simulink model "trajgen_pos_raspberrypi"  (R2018b)
settings: Solver=FixedStepDiscrete  StartTime=0.0  StopTime=10.0  RelTol=1e-3  EnableMultiTasking=on
settings Model: Creator=ihout_000  LastModifiedBy=ihout
settings SolverCC: PositivePriorityOrder=on
settings DataIOCC: LimitDataPoints=on  SaveFormat=Array
settings OptimizationCC: EnhancedBackFolding=on  PassReuseOutputArgsAs=Individual arguments  ExpressionDepthLimit=2147483647  MaxStackSize=64  SimCompilerOptimization=on  OptimizeBlockOrder=speed  DifferentSizesBufferReuse=on  OptimizationCustomize=off
settings DebuggingCC: UnderspecifiedInitializationDetection=Classic  MergeDetectMultiDrivingBlocksExec=none  SolverPrmCheckMsg=warning  ParameterTunabilityLossMsg=error  StateNameClashWarn=warning  SFUnexpectedBacktrackingDiag=warning  SFNoUnconditionalDefaultTransitionDiag=warning  SFExecutionAtInitializationDiag=none
settings HardwareCC: ProdBitPerPointer=32  ProdBitPerSizeT=32  ProdBitPerPtrDiffT=32  ProdLargestAtomicInteger=Long  ProdLargestAtomicFloat=Double  ProdWordSize=32  ProdHWDeviceType=ARM Compatible->ARM Cortex  UseEmbeddedCoderFeatures=off  UseSimulinkCoderFeatures=off
settings ModelReferenceCC: PropagateSignalLabelsOutOfModel=off
settings SFSimCC: SimUserIncludeDirs=ReflexxesTypeII\include\  SimUseLocalCustomCode=off  MATLABDynamicMemAlloc=off
settings SFSimCC: SimUserSources=|
  | ReflexxesTypeII\src\TypeIIRML\ReflexxesAPI.cpp
  | ReflexxesTypeII\src\TypeIIRML\TypeIIRMLCalculatePositionalExtrems.cpp
  | ReflexxesTypeII\src\TypeIIRML\TypeIIRMLDecisions.cpp
  | ReflexxesTypeII\src\TypeIIRML\TypeIIRMLDecisionTree1A.cpp
  | ReflexxesTypeII\src\TypeIIRML\TypeIIRMLDecisionTree1B.cpp
  | ReflexxesTypeII\src\TypeIIRML\TypeIIRMLDecisionTree1C.cpp
  | ReflexxesTypeII\src\TypeIIRML\TypeIIRMLDecisionTree2.cpp
  | ReflexxesTypeII\src\TypeIIRML\TypeIIRMLFallBackStrategy.cpp
  | ReflexxesTypeII\src\TypeIIRML\TypeIIRMLIsPhaseSynchronizationPossible.cpp
  | ReflexxesTypeII\src\TypeIIRML\TypeIIRMLPolynomial.cpp
  | ReflexxesTypeII\src\TypeIIRML\TypeIIRMLPosition.cpp
  | ReflexxesTypeII\src\TypeIIRML\TypeIIRMLQuicksort.cpp
  | ReflexxesTypeII\src\TypeIIRML\TypeIIRMLSetupModifiedSelectionVector.cpp
  | ReflexxesTypeII\src\TypeIIRML\TypeIIRMLStep1.cpp
  | ReflexxesTypeII\src\TypeIIRML\TypeIIRMLStep1IntermediateProfiles.cpp
  | ReflexxesTypeII\src\TypeIIRML\TypeIIRMLStep1Profiles.cpp
  | ReflexxesTypeII\src\TypeIIRML\TypeIIRMLStep2.cpp
  | ReflexxesTypeII\src\TypeIIRML\TypeIIRMLStep2IntermediateProfiles.cpp
  | ReflexxesTypeII\src\TypeIIRML\TypeIIRMLStep2PhaseSynchronization.cpp
  | ReflexxesTypeII\src\TypeIIRML\TypeIIRMLStep2Profiles.cpp
  | ReflexxesTypeII\src\TypeIIRML\TypeIIRMLStep2WithoutSynchronization.cpp
  | ReflexxesTypeII\src\TypeIIRML\TypeIIRMLStep3.cpp
  | ReflexxesTypeII\src\TypeIIRML\TypeIIRMLVelocity.cpp
  | ReflexxesTypeII\src\TypeIIRML\TypeIIRMLVelocityCalculatePositionalExtrems.cpp
  | ReflexxesTypeII\src\TypeIIRML\TypeIIRMLVelocityFallBackStrategy.cpp
  | ReflexxesTypeII\src\TypeIIRML\TypeIIRMLVelocityIsPhaseSynchronizationPossible.cpp
  | ReflexxesTypeII\src\TypeIIRML\TypeIIRMLVelocityMethods.cpp
  | ReflexxesTypeII\src\TypeIIRML\TypeIIRMLVelocitySetupPhaseSyncSelectionVector.cpp
settings RTWCC: SystemTargetFile=ert.tlc  HardwareBoard=Raspberry Pi  TLCOptions="-aInlineSetEventsForThisBaseRateFcn=TLC_FALSE -aSuppressMultiTaskScheduler=TLC_FALSE  -aRateBasedStepFcn=0"  TemplateMakefile=ert_default_tmf  GenerateReport=on  RTWUseLocalCustomCode=off  CustomInclude=ReflexxesTypeII\include\  Toolchain=GNU GCC Raspberry Pi  BuildConfiguration=Faster Runs  IncludeHyperlinkInReport=on  LaunchReport=on  TargetLang=C++  GenerateTraceInfo=on  GenerateTraceReport=on  GenerateTraceReportSl=on  GenerateTraceReportSf=on  GenerateTraceReportEml=on
settings RTWCC: CustomSource=|
  | ReflexxesTypeII\src\TypeIIRML\ReflexxesAPI.cpp
  | ReflexxesTypeII\src\TypeIIRML\TypeIIRMLCalculatePositionalExtrems.cpp
  | ReflexxesTypeII\src\TypeIIRML\TypeIIRMLDecisions.cpp
  | ReflexxesTypeII\src\TypeIIRML\TypeIIRMLDecisionTree1A.cpp
  | ReflexxesTypeII\src\TypeIIRML\TypeIIRMLDecisionTree1B.cpp
  | ReflexxesTypeII\src\TypeIIRML\TypeIIRMLDecisionTree1C.cpp
  | ReflexxesTypeII\src\TypeIIRML\TypeIIRMLDecisionTree2.cpp
  | ReflexxesTypeII\src\TypeIIRML\TypeIIRMLFallBackStrategy.cpp
  | ReflexxesTypeII\src\TypeIIRML\TypeIIRMLIsPhaseSynchronizationPossible.cpp
  | ReflexxesTypeII\src\TypeIIRML\TypeIIRMLPolynomial.cpp
  | ReflexxesTypeII\src\TypeIIRML\TypeIIRMLPosition.cpp
  | ReflexxesTypeII\src\TypeIIRML\TypeIIRMLQuicksort.cpp
  | ReflexxesTypeII\src\TypeIIRML\TypeIIRMLSetupModifiedSelectionVector.cpp
  | ReflexxesTypeII\src\TypeIIRML\TypeIIRMLStep1.cpp
  | ReflexxesTypeII\src\TypeIIRML\TypeIIRMLStep1IntermediateProfiles.cpp
  | ReflexxesTypeII\src\TypeIIRML\TypeIIRMLStep1Profiles.cpp
  | ReflexxesTypeII\src\TypeIIRML\TypeIIRMLStep2.cpp
  | ReflexxesTypeII\src\TypeIIRML\TypeIIRMLStep2IntermediateProfiles.cpp
  | ReflexxesTypeII\src\TypeIIRML\TypeIIRMLStep2PhaseSynchronization.cpp
  | ReflexxesTypeII\src\TypeIIRML\TypeIIRMLStep2Profiles.cpp
  | ReflexxesTypeII\src\TypeIIRML\TypeIIRMLStep2WithoutSynchronization.cpp
  | ReflexxesTypeII\src\TypeIIRML\TypeIIRMLStep3.cpp
  | ReflexxesTypeII\src\TypeIIRML\TypeIIRMLVelocity.cpp
  | ReflexxesTypeII\src\TypeIIRML\TypeIIRMLVelocityCalculatePositionalExtrems.cpp
  | ReflexxesTypeII\src\TypeIIRML\TypeIIRMLVelocityFallBackStrategy.cpp
  | ReflexxesTypeII\src\TypeIIRML\TypeIIRMLVelocityIsPhaseSynchronizationPossible.cpp
  | ReflexxesTypeII\src\TypeIIRML\TypeIIRMLVelocityMethods.cpp
  | ReflexxesTypeII\src\TypeIIRML\TypeIIRMLVelocitySetupPhaseSyncSelectionVector.cpp
settings CodeAppCC: ForceParamTrailComments=on  IgnoreCustomStorageClasses=off  OperatorAnnotations=on  SimulinkDataObjDesc=on  SFDataObjDesc=on  InsertBlockDesc=on
settings ERTTargetCC: MultiInstanceERTCode=on  CodeInterfacePackaging=C++ class  SupportNonInlinedSFcns=on  SupportVariableSizeSignals=on  RootIOFormat=Structure reference
settings ConfigComp: CovMetricSettings=dw  CovHtmlReporting=on  CovSaveCumulativeToWorkspaceVar=on  CovSaveSingleToWorkspaceVar=on  CovExternalEMLEnable=off

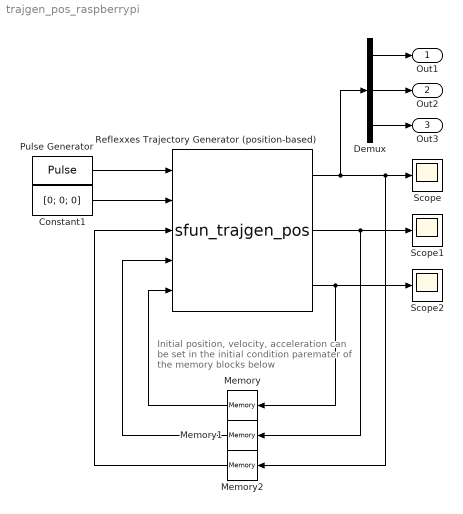
== system trajgen_pos_raspberrypi ==
  note: Initial position, velocity, acceleration
      | can be set in the initial condition
      | paremater of the memory blocks below
  Constant1 : Constant  Value=[0; 0; 0]
  Demux : Demux  Outputs=3
  Memory : Memory  InitialCondition=[0 0 0]
  Memory1 : Memory  InitialCondition=[0 0 0]
  Memory2 : Memory  InitialCondition=[2 -1 1]
  Pulse Generator : DiscretePulseGenerator  Amplitude=[10; 1; 5]  Period=500  PulseWidth=200  SampleTime=0.01
  Reflexxes Trajectory Generator (position-based) : S-Function  FunctionName=sfun_trajgen_pos  Parameters=ts,ndofs,vmax,amax,jmax,sync,final  SFunctionDeploymentMode=off  EnableBusSupport=off  mask{ts=1e-2, ndofs=3, vmax=[15 10 25], amax=[150 100 50], jmax=[500 1000 700], sync=PHASE_SYNCHRONIZATION_IF_POSSIBLE, final=KEEP_TARGET_VELOCITY}
      mask prompts: ts "Sample Time:"; ndofs "Number of DoF's:"; vmax "Maximum Velocity Vector:"; amax "Maximum Acceleration Vector:"; jmax "Maximum Jerk Vector:"; sync "Synchronization Behavior:"; final "After Final State Behavior:"
      mask TypeOptions sync: NO_SYNCHRONIZATION | PHASE_SYNCHRONIZATION_IF_POSSIBLE | ONLY_TIME_SYNCHRONIZATION | ONLY_PHASE_SYNCHRONIZATION
      mask TypeOptions final: KEEP_TARGET_VELOCITY | RECOMPUTE_TRAJECTORY
      mask Display:
      | port_label('input', 1, 'target_pos')
      | port_label('input', 2, 'target_vel')
      | port_label('input', 3, 'current_pos')
      | port_label('input', 4, 'current_vel')
      | port_label('input', 5, 'current_acc')
      | port_label('output', 1, 'pos')
      | port_label('output', 2, 'vel')
      | port_label('output', 3, 'acc')
  Scope : Scope
  Scope1 : Scope
  Scope2 : Scope
  Out1 : Outport
  Out2 : Outport  Port=2
  Out3 : Outport  Port=3
  wires:
  Pulse Generator/1 -> Reflexxes Trajectory Generator (position-based)/1
  Constant1/1 -> Reflexxes Trajectory Generator (position-based)/2
  Reflexxes Trajectory Generator (position-based)/1 -> Demux/1, Memory2/1, Scope/1
  Reflexxes Trajectory Generator (position-based)/2 -> Memory1/1, Scope1/1
  Reflexxes Trajectory Generator (position-based)/3 -> Scope2/1, Memory/1
  Demux/1 -> Out1/1
  Demux/2 -> Out2/1
  Demux/3 -> Out3/1
  Memory/1 -> Reflexxes Trajectory Generator (position-based)/5
  Memory1/1 -> Reflexxes Trajectory Generator (position-based)/4
  Memory2/1 -> Reflexxes Trajectory Generator (position-based)/3
